simulink model "P5_3"  (R2021a)
settings: Solver=VariableStepAuto  StartTime=0.0  StopTime=inf  RelTol=1e-3
libraries: instrumentseriallib x2
settings Model: Creator=escob  LastModifiedBy=ferna
settings SolverCC: AlgebraicLoopSolver=TrustRegion
settings DebuggingCC: SFMachineParentedDataDiag=warning

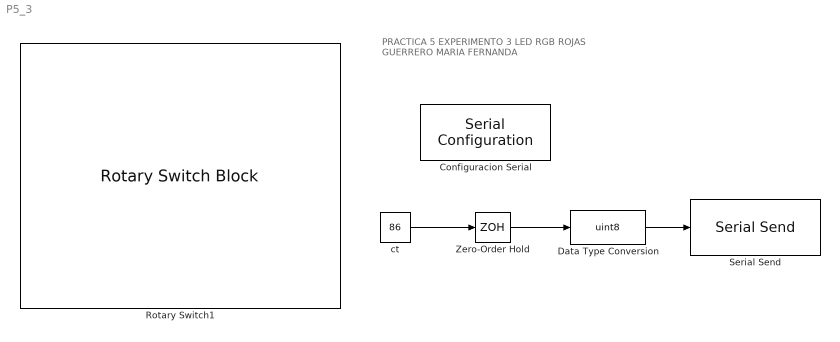
== system P5_3 ==
  note: PRACTICA 5 EXPERIMENTO 3 LED RGB
      | ROJAS GUERRERO MARIA FERNANDA
  Configuracion Serial : instrumentseriallib/Serial Configuration  Priority=-200000  Port=<Select a port...>  ComPort=<Select a port...>  BaudRate=9600  DataBits=8  Parity=none  StopBits=1  ByteOrder=little-endian  FlowControl=none  Timeout=10  SimulateUsing=Interpreted execution  BlockInModel=on
  "Data Type Conversion " : DataTypeConversion  OutDataTypeStr=uint8
  Rotary Switch1 : RotarySwitchBlock
      settings: Values={{'0%', '20%', '40%', '60%', '80%', '100%', 'ROJO', 'VERDE', 'AZUL'}, [1 20 40 60 80 100 82 86 65]}
  Serial Send : instrumentseriallib/Serial Send  Port=<Select a port...>  ComPort=<Select a port...>  Header=[]  Terminator=<none>  CustomTerminator=[]  EnableBlockingMode=on  SimulateUsing=Interpreted execution  BlockInModel=on
  Zero-Order Hold : ZeroOrderHold  SampleTime=0.5
  ct : Constant  Value=86
  wires:
  "Data Type Conversion "/1 -> Serial Send/1
  Zero-Order Hold/1 -> "Data Type Conversion "/1
  ct/1 -> Zero-Order Hold/1
